simulink model "w1p4"  (R2020a)
settings: Solver=VariableStepAuto  StartTime=0.0  StopTime=20  RelTol=1e-3
settings Model: Creator=akhil singh  LastModifiedBy=akhil singh

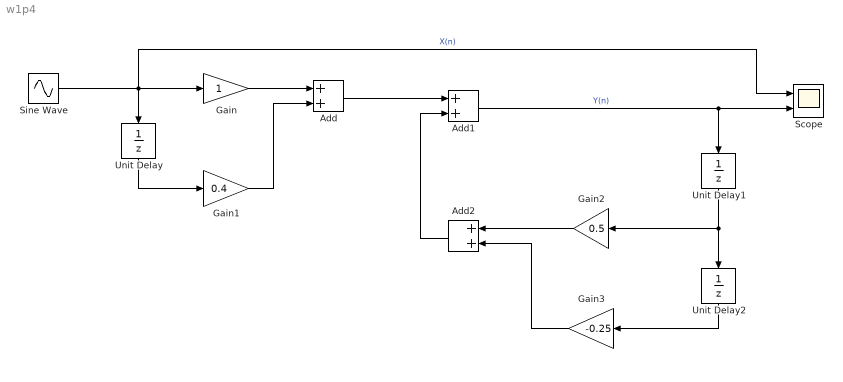
== system w1p4 ==
  Add : Sum
  Add1 : Sum
  Add2 : Sum
  Gain : Gain
  Gain1 : Gain  Gain=0.4
  Gain2 : Gain  Gain=0.5
  Gain3 : Gain  Gain=-0.25
  Scope : Scope  NumInputPorts=2
  Sine Wave : Sin  SampleTime=0
  Unit Delay : UnitDelay  SampleTime=-1  HasFrameUpgradeWarning=on
  Unit Delay1 : UnitDelay  SampleTime=-1  HasFrameUpgradeWarning=on
  Unit Delay2 : UnitDelay  SampleTime=-1  HasFrameUpgradeWarning=on
  wires:
  Sine Wave/1 -> Unit Delay/1, Gain/1, Scope/1  "X(n)"
  Unit Delay/1 -> Gain1/1
  Gain/1 -> Add/1
  Gain1/1 -> Add/2
  Add/1 -> Add1/1
  Add1/1 -> Unit Delay1/1, Scope/2  "Y(n)"
  Unit Delay1/1 -> Unit Delay2/1, Gain2/1
  Add2/1 -> Add1/2
  Gain2/1 -> Add2/1
  Unit Delay2/1 -> Gain3/1
  Gain3/1 -> Add2/2
